simulink model "MyControl_3SMCs_2022b_Ver"  (R2022b)
settings: Solver=FixedStepAuto  StartTime=0.0  StopTime=150  FixedStep=0.005  RelTol=1e-3
libraries: simulink x2, slpidlib x1
settings Model: Creator=Admin  LastModifiedBy=HIEU
settings SolverCC: AlgebraicLoopSolver=TrustRegion
settings DebuggingCC: ArithmeticOperatorsInVariantConditions=warning
settings SFSimCC: CustomCodeUndefinedFunction=UseInterfaceOnly

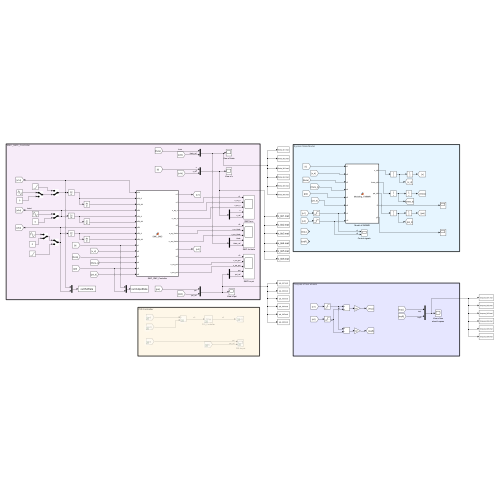
[thumbnail: Simulink's stored preview of the top-level diagram]
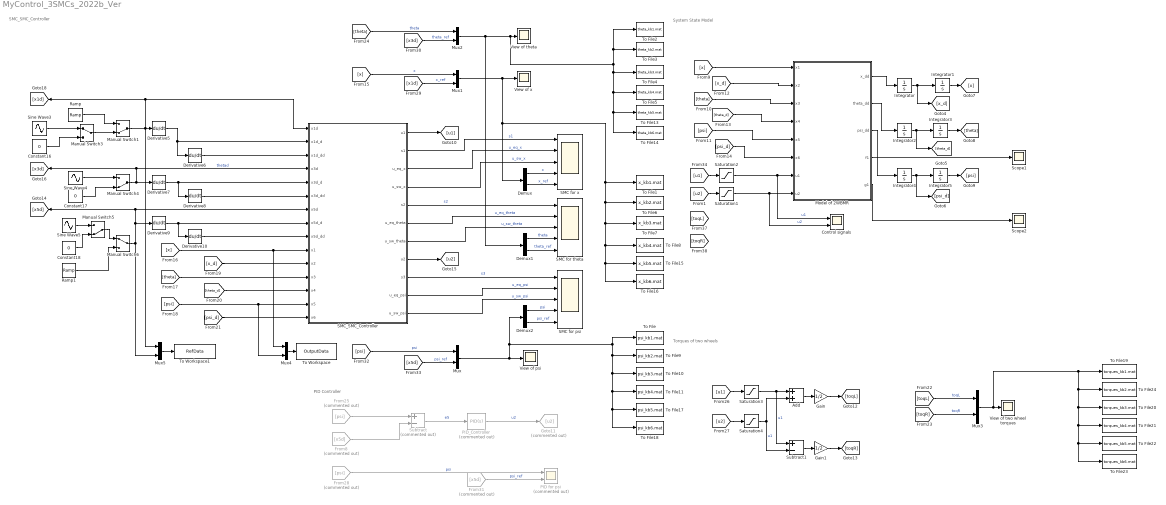
== system MyControl_3SMCs_2022b_Ver ==
  note: Torques of two wheels
  note: PID Controller
  note: System State Model
  note: SMC_SMC_Controller
  Add : Sum
  Constant16 : Constant  Value=0
  Constant17 : Constant  Value=0
  Constant18 : Constant  Value=0
  Control signals : Scope  NumInputPorts=2
  Demux : Demux  Outputs=2
  Demux1 : Demux  Outputs=2
  Demux2 : Demux  Outputs=2
  Derivative{5..10} (6 alike) : Derivative  CoefficientInTFapproximation=0.005
  From25 : From  Commented=on  GotoTag=psi
  From28 : From  Commented=on  GotoTag=psi
  From31 : From  Commented=on  GotoTag=x5d
  From8 : From  Commented=on  GotoTag=x5d
  Gain : Gain  Gain=1/2
  Gain1 : Gain  Gain=1/2
  Goto11 : Goto  Commented=on  GotoTag=u2
  Integrator{,1..2,4} (4 alike) : Integrator
  Integrator3 : Integrator  InitialCondition=pi/18*1
  Integrator5 : Integrator  InitialCondition=pi/18*0
  Manual Switch1 : ManualSwitch  CurrentSetting=0
  Manual Switch3 : ManualSwitch
  Manual Switch4 : ManualSwitch  CurrentSetting=0
  Manual Switch5 : ManualSwitch  CurrentSetting=0
  Manual Switch6 : ManualSwitch
  Model of 2WBMR : MATLAB Function  TreatAsAtomicUnit=on
  Mux{,1..5} (6 alike) : Mux  Inputs=2
  PID for psi : Scope  Commented=on  NumInputPorts=2
  PID_Controller : slpidlib/PID Controller  Commented=on  Controller=PID  Form=Ideal  TimeDomain=Continuous-time  UseExternalTs=off  SampleTime=-1  IntegratorMethod=Forward Euler  FilterMethod=Forward Euler  ControllerParametersSource=internal  P=9.0659  I=1/0.646  UseKiTs=off  D=0  N=100  UseFilter=on  TunerSelectOption=Transfer Function Based (PID Tuner App)  InitialConditionSource=internal  InitialConditionForIntegrator=0  InitialConditionForFilter=0  DifferentiatorICPrevScaledInput=0  ExternalReset=none  TrackingMode=off  Kt=1  LimitOutput=off  SatLimitsSource=internal  UpperSaturationLimit=inf  LowerSaturationLimit=-inf  LinearizeAsGain=on  AntiWindupMode=back-calculation  Kb=35  LimitIntegrator=off  UpperIntegratorSaturationLimit=inf  LowerIntegratorSaturationLimit=-inf  POutMin=[]  POutMax=[]  IOutMin=[]  IOutMax=[]  DOutMin=[]  DOutMax=[]  NOutMin=[]  NOutMax=[]  SumOutMin=[]  SumOutMax=[]  SaturationOutMin=[]  SaturationOutMax=[]  PParamMin=[]  PParamMax=[]  IParamMin=[]  IParamMax=[]  DParamMin=[]  DParamMax=[]  NParamMin=[]  NParamMax=[]  KbParamMin=[]  KbParamMax=[]  KtParamMin=[]  KtParamMax=[]  KbOutMin=[]  KbOutMax=[]  KtOutMin=[]  KtOutMax=[]  IntegratorOutMin=[]  IntegratorOutMax=[]  FilterOutMin=[]  FilterOutMax=[]  SumI1OutMin=[]  SumI1OutMax=[]  SumI2OutMin=[]  SumI2OutMax=[]  SumI3OutMin=[]  SumI3OutMax=[]  SumI4OutMin=[]  SumI4OutMax=[]  SumDOutMin=[]  SumDOutMax=[]  DifferentiatorOutMin=[]  DifferentiatorOutMax=[]  FilterDiffOutCoefMin=[]  FilterDiffOutCoefMax=[]  ReciprocalOutMin=[]  ReciprocalOutMax=[]  SumDenOutMin=[]  SumDenOutMax=[]  SumNumOutMin=[]  SumNumOutMax=[]  DivideOutMin=[]  DivideOutMax=[]  UdiffTsProdOutMin=[]  UdiffTsProdOutMax=[]  NTsProdOutMin=[]  NTsProdOutMax=[]  UintegralTsProdOutMin=[]  UintegralTsProdOutMax=[]  UngainTsProdOutMin=[]  UngainTsProdOutMax=[]  IntegratorContinuousStateAttributes=''  IntegratorStateMustResolveToSignalObject=off  IntegratorRTWStateStorageClass=Auto  FilterContinuousStateAttributes=''  FilterStateMustResolveToSignalObject=off  FilterRTWStateStorageClass=Auto  ParallelPVariant=Passthrough  IdealPVariant=InternalParameters  IVariant=InternalParameters  DVariant=InternalParameters  IntegratorVariant=Continuous  SatVariant=Disabled  AWVariant=Passthrough  PCopyVariant=Disabled  TRVariant=Disabled  FdbkBlocksVariant=Forward  IdealPFdbkVariant=Disabled  SatFdbkVariant=Disabled  DerivativeFilterVariant=ContFilter  NVariant=InternalParameters  NCopyVariant=Disabled  FilterICVariant=InternalICsFilter  IntegratorICVariant=InternalICs  ExternalResetVariant=Disabled  TRSumVariant=Passthrough  SumFdbkVariant=Disabled  SumVariant=Sum_PID  TsampFilterVariant=InternalTs  TsampNgainVariant=Passthrough  TsampIntegralVariant=Disabled_SignalSpec  ExternalSaturationOutDataTypeStr=Inherit: Same as second input
  Ramp : simulink/Sources/Ramp  slope=pi/40  start=0  InitialOutput=0
  Ramp1 : simulink/Sources/Ramp  slope=pi/40  start=0  InitialOutput=0
  SMC for psi : Scope  NumInputPorts=5
  SMC for theta : Scope  NumInputPorts=5
  SMC for x : Scope  NumInputPorts=5
  SMC_SMC_Controller : MATLAB Function  TreatAsAtomicUnit=on
  Saturation{1..4} (4 alike) : Saturate  UpperLimit=25  LowerLimit=-25
  Scope1 : Scope
  Scope2 : Scope
  Sine Wave3 : Sin  Amplitude=4  Frequency=0.1  SampleTime=0
  Sine Wave4 : Sin  SampleTime=0
  Sine Wave5 : Sin  Amplitude=pi/2  Frequency=0.1  SampleTime=0
  Subtract : Sum  Commented=on  Inputs=+-
  Subtract1 : Sum  Inputs=+-
  To File : ToFile  Filename=psi_kb1.mat  MatrixName=psi_kb1
  To File1 : ToFile  Filename=x_kb1.mat  MatrixName=x_kb1
  To File10 : ToFile  Filename=psi_kb3.mat  MatrixName=psi_kb3
  To File11 : ToFile  Filename=psi_kb4.mat  MatrixName=psi_kb4
  To File13 : ToFile  Filename=theta_kb5.mat  MatrixName=theta_kb5
  To File14 : ToFile  Filename=theta_kb6.mat  MatrixName=theta_kb6
  To File15 : ToFile  Filename=x_kb5.mat  MatrixName=x_kb5
  To File16 : ToFile  Filename=x_kb6.mat  MatrixName=x_kb6
  To File17 : ToFile  Filename=psi_kb5.mat  MatrixName=psi_kb5
  To File18 : ToFile  Filename=psi_kb6.mat  MatrixName=psi_kb6
  To File19 : ToFile  Filename=torques_kb1.mat  MatrixName=torques_kb1
  To File2 : ToFile  Filename=theta_kb1.mat  MatrixName=theta_kb1
  To File20 : ToFile  Filename=torques_kb3.mat  MatrixName=torques_kb3
  To File21 : ToFile  Filename=torques_kb4.mat  MatrixName=torques_kb4
  To File22 : ToFile  Filename=torques_kb5.mat  MatrixName=torques_kb5
  To File23 : ToFile  Filename=torques_kb6.mat  MatrixName=torques_kb6
  To File24 : ToFile  Filename=torques_kb2.mat  MatrixName=torques_kb2
  To File3 : ToFile  Filename=theta_kb2.mat  MatrixName=theta_kb2
  To File4 : ToFile  Filename=theta_kb3.mat  MatrixName=theta_kb3
  To File5 : ToFile  Filename=theta_kb4.mat  MatrixName=theta_kb4
  To File6 : ToFile  Filename=x_kb2.mat  MatrixName=x_kb2
  To File7 : ToFile  Filename=x_kb3.mat  MatrixName=x_kb3
  To File8 : ToFile  Filename=x_kb4.mat  MatrixName=x_kb4
  To File9 : ToFile  Filename=psi_kb2.mat  MatrixName=psi_kb2
  To Workspace : ToWorkspace  VariableName=OutputData  SampleTime=-1
  To Workspace1 : ToWorkspace  VariableName=RefData  SampleTime=-1
  View of psi : Scope
  View of theta : Scope
  View of two wheel torques : Scope
  View of x : Scope
  wires:
  Integrator3/1 -> [theta]
  Integrator/1 -> Integrator1/1, [x_d]
  Integrator2/1 -> Integrator3/1, [theta_d]
  Integrator1/1 -> [x]
  Integrator5/1 -> [psi]
  Integrator4/1 -> [psi_d], Integrator5/1
  Model of 2WBMR/1(x_dd) -> Integrator/1
  Model of 2WBMR/2(theta_dd) -> Integrator2/1
  Model of 2WBMR/3(psi_dd) -> Integrator4/1
  [theta] -> Mux2/1  "theta"
  [x_d] -> Model of 2WBMR/2(x2)
  [psi_d] -> Model of 2WBMR/6(x6)
  [psi] -> Model of 2WBMR/5(x5)
  [theta_d] -> Model of 2WBMR/4(x4)
  [theta] -> Model of 2WBMR/3(x3)
  [x] -> Model of 2WBMR/1(x1)
  Model of 2WBMR/4(f1) -> Scope1/1
  Model of 2WBMR/5(g1) -> Scope2/1
  [u2] -> Saturation1/1
  [x] -> Mux1/1  "x"
  [psi_d] -> SMC_SMC_Controller/15(x6)
  [psi] -> Mux4/2, SMC_SMC_Controller/14(x5)
  [theta_d] -> SMC_SMC_Controller/13(x4)
  [theta] -> SMC_SMC_Controller/12(x3)
  [x_d] -> SMC_SMC_Controller/11(x2)
  [x] -> Mux4/1, SMC_SMC_Controller/10(x1)
  Constant18/1 -> Manual Switch5/2
  Manual Switch5/1 -> Manual Switch6/1
  Sine Wave5/1 -> Manual Switch5/1
  Derivative9/1 -> Derivative10/1, SMC_SMC_Controller/8(x5d_d)
  Constant17/1 -> Manual Switch4/2
  Manual Switch4/1 -> Derivative7/1, SMC_SMC_Controller/4(x3d), [x3d]  "thetad"
  Derivative8/1 -> SMC_SMC_Controller/6(x3d_dd)
  Sine Wave4/1 -> Manual Switch4/1
  Derivative7/1 -> Derivative8/1, SMC_SMC_Controller/5(x3d_d)
  Constant16/1 -> Manual Switch3/2
  Derivative6/1 -> SMC_SMC_Controller/3(x1d_dd)
  Sine Wave3/1 -> Manual Switch3/1
  Derivative5/1 -> Derivative6/1, SMC_SMC_Controller/2(x1d_d)
  Gain1/1 -> [toqR]
  Gain/1 -> [toqL]
  SMC_SMC_Controller/1(u1) -> [u1]
  [toqR] -> Mux3/2  "toqR"
  From8/1 -> Subtract/2
  Subtract/1 -> PID_Controller/1  "e5"
  PID_Controller/1 -> Goto11/1  "u2"
  [u1] -> Saturation3/1
  [u2] -> Saturation4/1
  Add/1 -> Gain/1
  Subtract1/1 -> Gain1/1
  From28/1 -> PID for psi/1  "psi"
  [x1d] -> Mux1/2  "x_ref"
  From31/1 -> PID for psi/2  "psi_ref"
  [x3d] -> Mux2/2  "theta_ref"
  Saturation1/1 -> Control signals/2, Model of 2WBMR/8(u2)  "u2"
  SMC_SMC_Controller/2(s1) -> SMC for x/1  "s1"
  SMC_SMC_Controller/5(s2) -> SMC for theta/1  "s2"
  SMC_SMC_Controller/3(u_eq_x) -> SMC for x/2  "u_eq_x"
  SMC_SMC_Controller/4(u_sw_x) -> SMC for x/3  "u_sw_x"
  Mux1/1 -> To File1/1, To File6/1, To File7/1, To File8/1, To File15/1, To File16/1, Demux/1, View of x/1
  Mux2/1 -> View of theta/1, To File2/1, To File3/1, To File14/1, To File13/1, To File5/1, To File4/1, Demux1/1
  SMC_SMC_Controller/6(u_eq_theta) -> SMC for theta/2  "u_eq_theta"
  SMC_SMC_Controller/7(u_sw_theta) -> SMC for theta/3  "u_sw_theta"
  Demux/1 -> SMC for x/4  "x"
  Demux1/1 -> SMC for theta/4  "theta"
  Demux1/2 -> SMC for theta/5  "theta_ref"
  Demux/2 -> SMC for x/5  "x_ref"
  [u1] -> Saturation2/1
  Saturation2/1 -> Control signals/1, Model of 2WBMR/7(u1)  "u1"
  [toqL] -> Mux3/1  "toqL"
  Ramp1/1 -> Manual Switch6/2
  Manual Switch6/1 -> Mux5/2, Derivative9/1, [x5d], SMC_SMC_Controller/7(x5d)
  From25/1 -> Subtract/1
  Derivative10/1 -> SMC_SMC_Controller/9(x5d_dd)
  SMC_SMC_Controller/8(u2) -> [u2]
  SMC_SMC_Controller/9(s3) -> SMC for psi/1  "s3"
  SMC_SMC_Controller/10(u_eq_psi) -> SMC for psi/2  "u_eq_psi"
  SMC_SMC_Controller/11(u_sw_psi) -> SMC for psi/3  "u_sw_psi"
  [x5d] -> Mux/2  "psi_ref"
  [psi] -> Mux/1  "psi"
  Demux2/1 -> SMC for psi/4  "psi"
  Demux2/2 -> SMC for psi/5  "psi_ref"
  Mux/1 -> Demux2/1, To File18/1, To File17/1, To File11/1, To File10/1, To File9/1, To File/1, View of psi/1
  Saturation3/1 -> Subtract1/1, Add/1  "u1"
  Saturation4/1 -> Add/2, Subtract1/2  "u1"
  Mux3/1 -> To File24/1, To File20/1, To File21/1, To File22/1, To File23/1, To File19/1, View of two wheel torques/1
  Manual Switch1/1 -> Mux5/1, Derivative5/1, SMC_SMC_Controller/1(x1d), [x1d]
  Manual Switch3/1 -> Manual Switch1/2
  Ramp/1 -> Manual Switch1/1
  Mux4/1 -> To Workspace/1
  Mux5/1 -> To Workspace1/1

== matlab function MyControl_3SMCs_2022b_Ver/Model of 2WBMR ==
  data: x1 input; x_dd output; x2 input; x3 input; x4 input; x5 input; x6 input; u1 input; u2 input; theta_dd output; psi_dd output; f1 output; g1 output
function [x_dd,theta_dd,psi_dd, f1, g1] = Modeling_TWBMR(x1,x2,x3,x4,x5,x6,u1,u2)

%% Parameters
mB=21; %mass of body inverted pendulum   %21
mW=0.512; %mass of each wheel
J=1.35e-3; K=6.73e-4; %mass moment of inertia of each wheel 
r=0.0725; %radius of each wheel
g=9.81; %gravity
d=0.59; %distance between two wheels
l=0.6; %length of inverted pendulum
I1 = 1.476; I2=2.624; I3=1.476; %mass moment of inertia of each wheel
alpha=0.5; % damping torque

%% Model

% x_dd = (r^2*(mB*l^2 + I2)*(x4*((2*alpha)/r + l*mB*x4*sin(x3)) - (2*alpha*x2)/r^2 + l*mB*x6^2*sin(x3)))/(l^2*mB^2*r^2 + 2*mW*l^2*mB*r^2 + 2*J*l^2*mB - 12*cos(x3)*l*mB*r^2 + I2*mB*r^2 + 2*I2*mW*r^2 + 2*I2*J) + (r*u1*(mB*l^2 + I2))/(l^2*mB^2*r^2 + 2*mW*l^2*mB*r^2 + 2*J*l^2*mB - 12*cos(x3)*l*mB*r^2 + I2*mB*r^2 + 2*I2*mW*r^2 + 2*I2*J) + (l*mB*r^2*u1*cos(x3))/(l^2*mB^2*r^2 + 2*mW*l^2*mB*r^2 + 2*J*l^2*mB - 12*cos(x3)*l*mB*r^2 + I2*mB*r^2 + 2*I2*mW*r^2 + 2*I2*J) - (l*mB*r^2*cos(x3)*(cos(x3)*sin(x3)*(mB*l^2 + I1 - I3)*x6^2 - 2*alpha*x4 + (2*alpha*x2)/r + g*l*mB*sin(x3)))/(l^2*mB^2*r^2 + 2*mW*l^2*mB*r^2 + 2*J*l^2*mB - 12*cos(x3)*l*mB*r^2 + I2*mB*r^2 + 2*I2*mW*r^2 + 2*I2*J);
% theta_dd = ((2*J + mB*r^2 + 2*mW*r^2)*(cos(x3)*sin(x3)*(mB*l^2 + I1 - I3)*x6^2 - 2*alpha*x4 + (2*alpha*x2)/r + g*l*mB*sin(x3)))/(l^2*mB^2*r^2 + 2*mW*l^2*mB*r^2 + 2*J*l^2*mB - 12*cos(x3)*l*mB*r^2 + I2*mB*r^2 + 2*I2*mW*r^2 + 2*I2*J) - (12*r*u1)/(l^2*mB^2*r^2 + 2*mW*l^2*mB*r^2 + 2*J*l^2*mB - 12*cos(x3)*l*mB*r^2 + I2*mB*r^2 + 2*I2*mW*r^2 + 2*I2*J) - (u1*(2*J + mB*r^2 + 2*mW*r^2))/(l^2*mB^2*r^2 + 2*mW*l^2*mB*r^2 + 2*J*l^2*mB - 12*cos(x3)*l*mB*r^2 + I2*mB*r^2 + 2*I2*mW*r^2 + 2*I2*J) - (12*r^2*(x4*((2*alpha)/r + l*mB*x4*sin(x3)) - (2*alpha*x2)/r^2 + l*mB*x6^2*sin(x3)))/(l^2*mB^2*r^2 + 2*mW*l^2*mB*r^2 + 2*J*l^2*mB - 12*cos(x3)*l*mB*r^2 + I2*mB*r^2 + 2*I2*mW*r^2 + 2*I2*J);
% psi_dd = - (r^2*(x6*((alpha*d^2)/(2*r^2) + x4*cos(x3)*sin(x3)*(mB*l^2 + I1 - I3)) + l*mB*x2*x6*sin(x3) + x4*x6*cos(x3)*sin(x3)*(mB*l^2 + I1 - I3)))/(J*d^2 + I3*r^2 + 2*K*r^2 + d^2*mW*r^2 + I1*r^2*sin(x3)^2 - I3*r^2*sin(x3)^2 + l^2*mB*r^2*sin(x3)^2) - (d*r*u2)/(2*(J*d^2 + I3*r^2 + 2*K*r^2 + d^2*mW*r^2 + I1*r^2*sin(x3)^2 - I3*r^2*sin(x3)^2 + l^2*mB*r^2*sin(x3)^2));


a11 = mB + 2*mW + 2*J/r^2;
a12 = mB*l*cos(x3);
a21 = a12;
a22 = I2+mB*l*l;
a33 = I3 + 2*K + (mW + J/r/r)*(d^2)/2 - (I3 - I1 - mB*l*l)*sin(x3)^2;

c12 = -mB*l*x4*sin(x3);
c13 = -mB*l*x6*sin(x3);
c23 = (I3-I1-mB*l*l)*x6*sin(x3)*cos(x3);
c31 = mB*l*x6*sin(x3);
c32 = -(I3-I1-mB*l*l)*x6*sin(x3)*cos(x3);
c33 = -(I3-I1-mB*l*l)*x4*sin(x3)*cos(x3);

d11 = 2*alpha/r^2;
d22 = 2*alpha;
d12 = -d22/r;
d21 = d12;
d33 = d^2/(2*r^2)*alpha;

% M*q_dd + (C+D)*q_d + G = Bto
% q_dd = M^-1 * (Bto - G - (C+D)*q_d )

M = [a11 a12 0;
     a21 a22 0; 
     0   0   a33];
C = [0   c12 c13; 
     0   0   c23; 
     c31 c32 c33];
D = [d11 d12 0;
     d21 d22 0;
     0   0   d33];
q = [x1; x3; x5];
q_d = [x2; x4; x6];
G = [0; -mB*l*g*sin(x3); 0];
Z = [1/r 0  0
     0 -1 0
     0 0  -d/(2*r)];

% B=[u1; u2; u3];

Fx = -inv(M)*(G+C*q_d+D*q_d);
f1 = Fx(1);
f2 = Fx(2);
f3 = Fx(3);

Gx = inv(M) * Z;
g1 = Gx(1) + Gx(4);
g2 = Gx(2) + Gx(5);
g3 = Gx(9);



x_dd = f1 + g1 * u1;
theta_dd = f2 + g2 * u1;
psi_dd = f3 + g3 * u2;

== matlab function MyControl_3SMCs_2022b_Ver/SMC_SMC_Controller ==
  settings: updateMethod=DISCRETE  sampleTime=0.005
  data: x1d input; u1 output; s1 output; u_eq_x output; u_sw_x output; s2 output; x1d_d input; x1d_dd input; x3d input; x3d_d input; x3d_dd input; x5d input; x5d_d input; x5d_dd input; x1 input; x2 input; x3 input; x4 input; x5 input; x6 input; u_eq_theta output; u_sw_theta output; u2 output; s3 output; u_eq_psi output; u_sw_psi output
function [u1, s1, u_eq_x, u_sw_x, s2, u_eq_theta, u_sw_theta, u2, s3, u_eq_psi, u_sw_psi]  = SMC_SMC(x1d, x1d_d, x1d_dd, x3d, x3d_d, x3d_dd, x5d, x5d_d, x5d_dd, x1, x2, x3, x4, x5, x6)
    %% Parameters
    mB = 21;      % mass of Pendulum Body     %21
    mW = 0.512;       % mass of each wheel
    J = 1.35e-3; K = 6.73e-4;     % mass moment of inertia of each wheel
    r = 0.0725;      % radius of wheels
    g = 9.81;     % gravity
    d = 0.45;     % distance between the two wheels
    l = 0.6;     % length of pendulum
    I1 = 1.476; I2 = 2.624; I3 = 1.476;       % mass moment of inertia of the pendulum body
    alpha = 0.5;      % damping torque
    
    
    a11 = mB + 2*mW + 2*J/r^2;
    a12 = mB*l*cos(x3);
    a21 = a12;
    a22 = I2+mB*l*l;
    a33 = I3 + 2*K + (mW + J/r/r)*(d^2)/2 - (I3 - I1 - mB*l*l)*sin(x3)^2;
    
    c12 = -mB*l*x4*sin(x3);
    c13 = -mB*l*x6*sin(x3);
    c23 = (I3-I1-mB*l*l)*x6*sin(x3)*cos(x3);
    c31 = mB*l*x6*sin(x3);
    c32 = -(I3-I1-mB*l*l)*x6*sin(x3)*cos(x3);
    c33 = -(I3-I1-mB*l*l)*x4*sin(x3)*cos(x3);
    
    d11 = 2*alpha/r^2;
    d22 = 2*alpha;
    d12 = -d22/r;
    d21 = d12;
    d33 = (d^2/(2*r^2))*alpha;
    
    M = [a11 a12 0;
         a21 a22 0; 
         0   0   a33];
    C = [0   c12 c13; 
         0   0   c23; 
         c31 c32 c33];
    D = [d11 d12 0;
         d21 d22 0;
         0   0   d33];
    q = [x1; x3; x5];
    q_d = [x2; x4; x6];
    G = [0; -mB*l*g*sin(x3); 0];
    Z = [1/r 0  0
         0 -1 0
         0 0  -d/(2*r)];
    
    Fx = -inv(M)*(G+C*q_d+D*q_d);
    f1 = Fx(1);
    f2 = Fx(2);
    f3 = Fx(3);

    Gx = inv(M) * Z;
    g1 = Gx(1) + Gx(4);
    g2 = Gx(2) + Gx(5);
    g3 = Gx(9);

    %% Control parameters
    % First SMC controlling x
    a1 = 140; 
    beta1 = 0.1;
    k1 = 1;
    
    % Second SMC controlling theta
    a2 = 250;
    beta2 = 0.1;
    k2 = 5;
    
    % Third SMC controlling psi
    a3 = 2.5; %25;
    beta3 = 0.01;
    k3 = 3; %15;

    
    %% Sliding surfaces
    e1 = -(x1 - x1d);
    e2 = -(x2 - x1d_d);
    e3 = (x3 - x3d);
    e4 = (x4 - x3d_d);
    e5 = (x5 - x5d);
    e6 = (x6 - x5d_d);
    
    s1 = a1*e1 + e2;
    s2 = a2*e3 + e4;
    s3 = a3*e5 + e6;

    %% Outputs
    u_x = (1/g1)*(-a1*e2 - f1 + x1d_dd - beta1*sign(s1)-k1*s1);
    u_eq_x = (1/g1)*(-a1*e2 - f1 + x1d_dd);
    u_sw_x = (1/g1)*(- beta1*sign(s1)-k1*s1);

    u_theta = (1/g2)*(-a2*e4 - f2 + x3d_dd - beta2*sign(s2)-k2*s2);
    u_eq_theta = (1/g2)*(-a2*e4 - f2 + x3d_dd);
    u_sw_theta = (1/g2)*(- beta2*sign(s2)-k2*s2);

    u_psi = (1/g3)*(-a3*e6 - f3 + x5d_dd - beta3*sign(s3)-k3*s3);
    u_eq_psi = (1/g3)*(-a3*e6 - f3 + x5d_dd);
    u_sw_psi = (1/g3)*(- beta3*sign(s3)-k3*s3);

    u1 = u_x + u_theta;
    u2 = u_psi;
end

function y = sat(x)
    if x > 1
        y = 1;
    elseif x < -1
        y = -1;
    else
        y = x;
    end
end
